simulink model "RmtAPP_ChkSig"  (R2016b)
settings: configuration reference "CodeGenConfigSet" (kept outside this file)
values from neighbouring files (symbols this model uses):
  RmtAPP_drLimNeg_C = Calibration.Parameter    [init_RmtAPP_ChkSig.m]    (also in init_RmtAPP_ChkSig_SIL.m = Simulink.Parameter)
  RmtAPP_drLimpMax_C = Calibration.Parameter    [init_RmtAPP_ChkSig.m]    (also in init_RmtAPP_ChkSig_SIL.m = Simulink.Parameter)
  RmtAPP_drLimPos_C = Calibration.Parameter    [init_RmtAPP_ChkSig.m]    (also in init_RmtAPP_ChkSig_SIL.m = Simulink.Parameter)
  RmtAPP_rLimpMax_C = Calibration.Parameter    [init_RmtAPP_ChkSig.m]    (also in init_RmtAPP_ChkSig_SIL.m = Simulink.Parameter)
  RmtAPP_rPlaMaxVal_C = Calibration.Parameter    [init_RmtAPP_ChkSig.m]    (also in init_RmtAPP_ChkSig_SIL.m = Simulink.Parameter)
  RmtAPP_rThresAliveDet_C = Calibration.Parameter    [init_RmtAPP_ChkSig.m]    (also in init_RmtAPP_ChkSig_SIL.m = Simulink.Parameter)
  RmtAPP_swtAliveDetEna_C = Calibration.Parameter    [init_RmtAPP_ChkSig.m]    (also in init_RmtAPP_ChkSig_SIL.m = Simulink.Parameter)
  RmtAPP_swtPlaChkEna_C = Calibration.Parameter    [init_RmtAPP_ChkSig.m]    (also in init_RmtAPP_ChkSig_SIL.m = Simulink.Parameter)
  RmtAPP_tiAliveDebHiLo_C = Calibration.Parameter    [init_RmtAPP_ChkSig.m]    (also in init_RmtAPP_ChkSig_SIL.m = Simulink.Parameter)
  RmtAPP_tiAliveDebLoHi_C = Calibration.Parameter    [init_RmtAPP_ChkSig.m]    (also in init_RmtAPP_ChkSig_SIL.m = Simulink.Parameter)
undefined symbols (not defined in the file or in its folder): RmtAPP_ChkSig_DT, Switch_conv
libraries: CXLib x9
settings Model: Creator=bianxuyin  LastModifiedBy=bianxuyin
settings ConfigSetRef: SourceLocation=Base Workspace

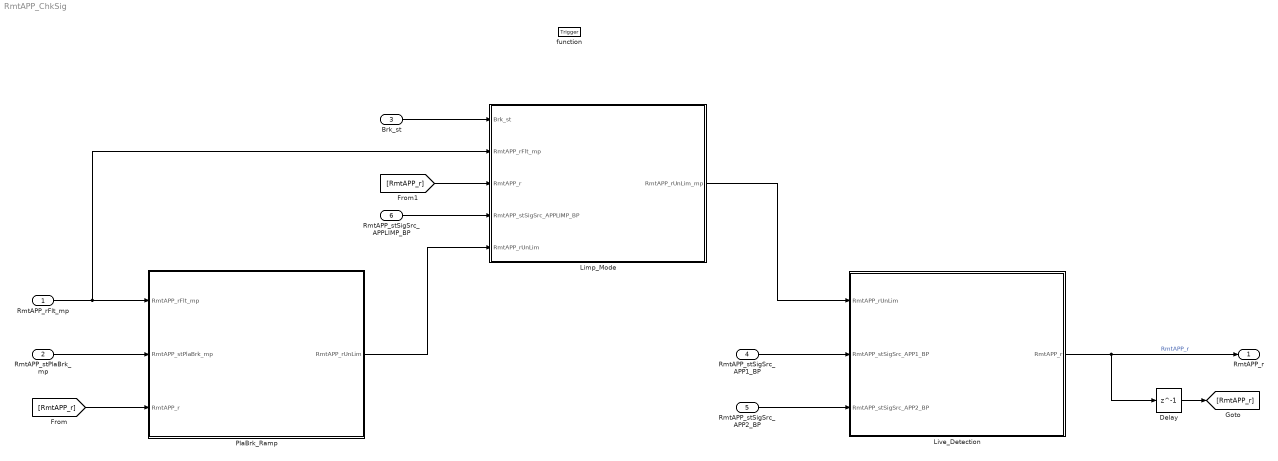
== system RmtAPP_ChkSig ==
  RmtAPP_rFlt_mp : Inport  Tag=%  Description=Remote Acceleration pedal position filtered value  OutMin=0  OutMax=100  OutDataTypeStr=Accpedal_rate
  RmtAPP_stPlaBrk_mp : Inport  Description=State of plausibility RmtAPP with brake  Port=2  OutMin=0  OutMax=1  OutDataTypeStr=boolean
  Brk_st : Inport  Description=Brake switch state  Port=3  OutMin=0  OutMax=255  OutDataTypeStr=State_uint8
  RmtAPP_stSigSrc_APP1_BP : Inport  Description=Sensor 1 is the reference variable, Sensor 2 value is defective  Port=4  OutMin=0  OutMax=1  OutDataTypeStr=boolean
  RmtAPP_stSigSrc_APP2_BP : Inport  Description=Sensor 2 is the reference variable,Sensor1 value is defective  Port=5  OutMin=0  OutMax=1  OutDataTypeStr=boolean
  RmtAPP_stSigSrc_APPLIMP_BP : Inport  Description=Substitute operation active, remote accelerator pedal sensor value and accelerator pedal sensor increase are limited  Port=6  OutMin=0  OutMax=1  OutDataTypeStr=boolean
  function : TriggerPort  TriggerType=function-call  VariantControl=Variant
  Delay : Delay  DelayLength=1  InitialCondition=0
  Limp_Mode : Subsystem
  Live_Detection : Subsystem
  PlaBrk_Ramp : Subsystem
  RmtAPP_r : Outport  Tag=%  Description=Remote Acceleration pedal sensor 1 value after fault handling  OutMin=0  OutMax=100  OutDataTypeStr=Accpedal_rate
  wires:
  Brk_st/1 -> Limp_Mode/1(Brk_st)
  RmtAPP_stSigSrc_APPLIMP_BP/1 -> Limp_Mode/4(RmtAPP_stSigSrc_APPLIMP_BP)
  Limp_Mode/1(RmtAPP_rUnLim_mp) -> Live_Detection/1(RmtAPP_rUnLim)
  RmtAPP_stSigSrc_APP1_BP/1 -> Live_Detection/2(RmtAPP_stSigSrc_APP1_BP)
  RmtAPP_stSigSrc_APP2_BP/1 -> Live_Detection/3(RmtAPP_stSigSrc_APP2_BP)
  Live_Detection/1(RmtAPP_r) -> Delay/1, RmtAPP_r/1  "RmtAPP_r"
  PlaBrk_Ramp/1(RmtAPP_rUnLim) -> Limp_Mode/5(RmtAPP_rUnLim)
  RmtAPP_rFlt_mp/1 -> Limp_Mode/2(RmtAPP_rFlt_mp), PlaBrk_Ramp/1(RmtAPP_rFlt_mp)
  RmtAPP_stPlaBrk_mp/1 -> PlaBrk_Ramp/2(RmtAPP_stPlaBrk_mp)
  Delay/1 -> [RmtAPP_r]
  [RmtAPP_r] -> PlaBrk_Ramp/3(RmtAPP_r)
  [RmtAPP_r] -> Limp_Mode/3(RmtAPP_r)

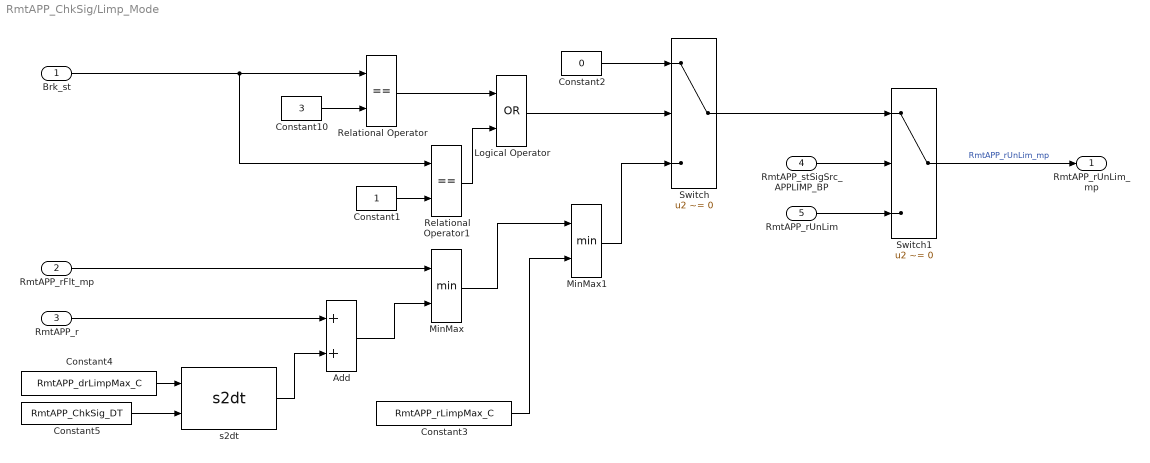
== system RmtAPP_ChkSig/Limp_Mode ==
  Brk_st : Inport  Description=Brake switch state  OutMin=0  OutMax=255
  RmtAPP_rFlt_mp : Inport  Tag=%  Description=Remote Acceleration pedal position filtered value  Port=2  OutMin=0  OutMax=100
  RmtAPP_r : Inport  Tag=%  Description=Remote Acceleration pedal position filtered value  Port=3  OutMin=0  OutMax=100
  RmtAPP_stSigSrc_APPLIMP_BP : Inport  Description=Substitute operation active, remote accelerator pedal sensor value and accelerator pedal sensor increase are limited  Port=4  OutMin=0  OutMax=1
  RmtAPP_rUnLim : Inport  Tag=%  Description=Remote Acceleration pedal position filtered value  Port=5  OutMin=0  OutMax=100
  Add : Sum  InputSameDT=on
  Constant1 : Constant  OutDataTypeStr=Inherit: Inherit via back propagation
  Constant10 : Constant  Value=3  OutDataTypeStr=Inherit: Inherit via back propagation
  Constant2 : Constant  Value=0  OutDataTypeStr=Inherit: Inherit via back propagation
  Constant3 : Constant  Value=RmtAPP_rLimpMax_C
  Constant4 : Constant  Value=RmtAPP_drLimpMax_C
  Constant5 : Constant  Value=RmtAPP_ChkSig_DT
  Logical Operator : Logic  Operator=OR  AllPortsSameDT=off  OutDataTypeStr=boolean
  MinMax : MinMax  Inputs=2  InputSameDT=on
  MinMax1 : MinMax  Inputs=2  InputSameDT=on
  Relational Operator : RelationalOperator  Operator===  OutDataTypeStr=boolean  RndMeth=Simplest
  Relational Operator1 : RelationalOperator  Operator===  OutDataTypeStr=boolean  RndMeth=Simplest
  Switch : Switch  Criteria=u2 ~= 0
  Switch1 : Switch  Criteria=u2 ~= 0
  s2dt : CXLib/s2dt
  RmtAPP_rUnLim_mp : Outport  Tag=%  Description=Remote Acceleration pedal sensor 1 value after fault handling  OutMin=0  OutMax=100  OutDataTypeStr=Accpedal_rate
  wires:
  Brk_st/1 -> Relational Operator1/1, Relational Operator/1
  Constant10/1 -> Relational Operator/2
  Relational Operator/1 -> Logical Operator/1
  Relational Operator1/1 -> Logical Operator/2
  Constant1/1 -> Relational Operator1/2
  Logical Operator/1 -> Switch/2
  Constant2/1 -> Switch/1
  MinMax/1 -> MinMax1/1
  MinMax1/1 -> Switch/3
  Constant3/1 -> MinMax1/2
  Add/1 -> MinMax/2
  RmtAPP_r/1 -> Add/1
  RmtAPP_rFlt_mp/1 -> MinMax/1
  s2dt/1 -> Add/2
  Constant4/1 -> s2dt/1
  Constant5/1 -> s2dt/2
  Switch/1 -> Switch1/1
  RmtAPP_stSigSrc_APPLIMP_BP/1 -> Switch1/2
  RmtAPP_rUnLim/1 -> Switch1/3
  Switch1/1 -> RmtAPP_rUnLim_mp/1  "RmtAPP_rUnLim_mp"

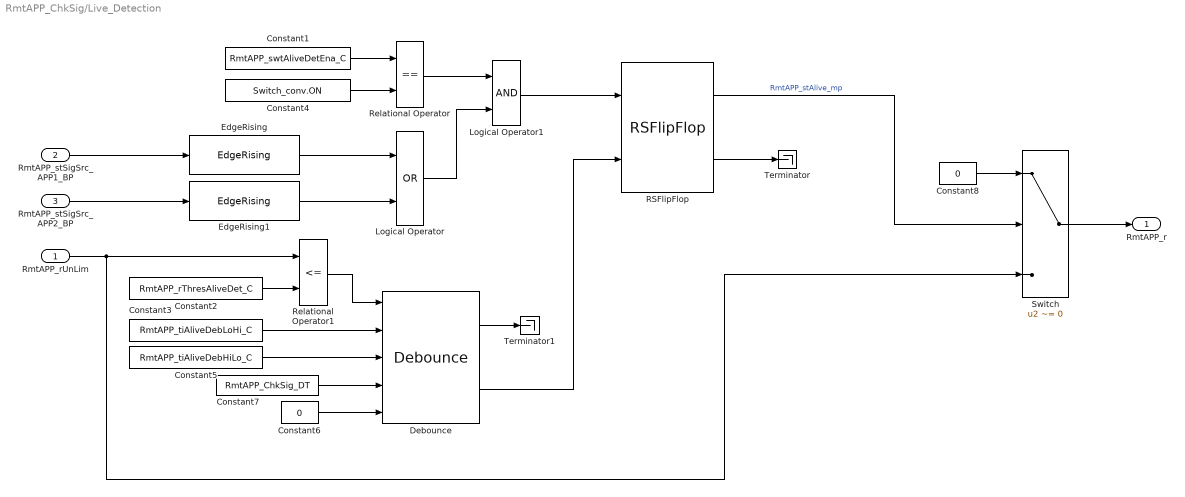
== system RmtAPP_ChkSig/Live_Detection ==
  RmtAPP_rUnLim : Inport  Description=Sensor 1 is the reference variable, Sensor 2 value is defective  OutMin=0  OutMax=1  OutDataTypeStr=Accpedal_rate
  RmtAPP_stSigSrc_APP1_BP : Inport  Description=Sensor 1 is the reference variable, Sensor 2 value is defective  Port=2  OutMin=0  OutMax=1  OutDataTypeStr=boolean
  RmtAPP_stSigSrc_APP2_BP : Inport  Description=Sensor 2 is the reference variable,Sensor1 value is defective  Port=3  OutMin=0  OutMax=1  OutDataTypeStr=boolean
  Constant1 : Constant  Value=RmtAPP_swtAliveDetEna_C
  Constant2 : Constant  Value=RmtAPP_rThresAliveDet_C
  Constant3 : Constant  Value=RmtAPP_tiAliveDebLoHi_C
  Constant4 : Constant  Value=Switch_conv.ON  OutDataTypeStr=Inherit: Inherit via back propagation
  Constant5 : Constant  Value=RmtAPP_tiAliveDebHiLo_C
  Constant6 : Constant  Value=0  OutDataTypeStr=Inherit: Inherit via back propagation
  Constant7 : Constant  Value=RmtAPP_ChkSig_DT  OutDataTypeStr=Inherit: Inherit via back propagation
  Constant8 : Constant  Value=0  OutDataTypeStr=Inherit: Inherit via back propagation
  Debounce : CXLib/Debounce
  EdgeRising : CXLib/EdgeRising
  EdgeRising1 : CXLib/EdgeRising
  Logical Operator : Logic  Operator=OR  OutDataTypeStr=boolean
  Logical Operator1 : Logic  OutDataTypeStr=boolean
  RSFlipFlop : CXLib/RSFlipFlop
  Relational Operator : RelationalOperator  Operator===  OutDataTypeStr=boolean  RndMeth=Simplest  InputSameDT=on
  Relational Operator1 : RelationalOperator  Operator=<=  OutDataTypeStr=boolean  RndMeth=Simplest  InputSameDT=on
  Switch : Switch  Criteria=u2 ~= 0
  Terminator : Terminator
  Terminator1 : Terminator
  RmtAPP_r : Outport  Tag=%  Description=Remote Acceleration pedal sensor 1 value after fault handling  OutMin=0  OutMax=100  OutDataTypeStr=Accpedal_rate
  wires:
  RmtAPP_stSigSrc_APP1_BP/1 -> EdgeRising/1
  Constant4/1 -> Relational Operator/2
  Constant1/1 -> Relational Operator/1
  Relational Operator/1 -> Logical Operator1/1
  Logical Operator/1 -> Logical Operator1/2
  Logical Operator1/1 -> RSFlipFlop/1
  RSFlipFlop/2 -> Terminator/1
  Debounce/1 -> Terminator1/1
  Debounce/2 -> RSFlipFlop/2
  Relational Operator1/1 -> Debounce/1
  RmtAPP_rUnLim/1 -> Relational Operator1/1, Switch/3
  Constant2/1 -> Relational Operator1/2
  Constant3/1 -> Debounce/2
  Constant5/1 -> Debounce/3
  Constant6/1 -> Debounce/5
  Constant7/1 -> Debounce/4
  RSFlipFlop/1 -> Switch/2  "RmtAPP_stAlive_mp"
  Constant8/1 -> Switch/1
  Switch/1 -> RmtAPP_r/1
  EdgeRising/1 -> Logical Operator/1
  RmtAPP_stSigSrc_APP2_BP/1 -> EdgeRising1/1
  EdgeRising1/1 -> Logical Operator/2

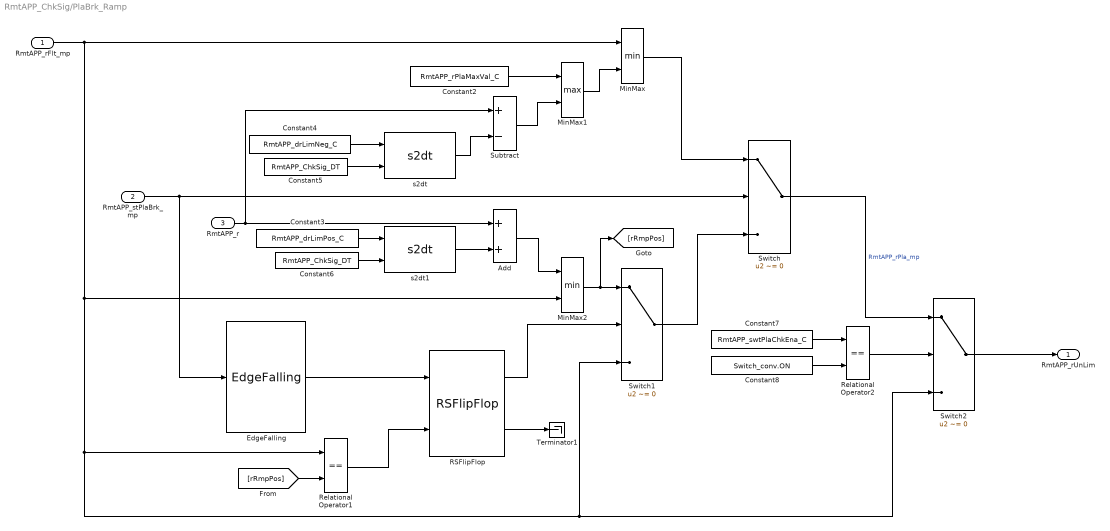
== system RmtAPP_ChkSig/PlaBrk_Ramp ==
  RmtAPP_rFlt_mp : Inport  Tag=%  Description=Remote Acceleration pedal position filtered value  OutMin=0  OutMax=100
  RmtAPP_stPlaBrk_mp : Inport  Description=State of plausibility RmtAPP with brake  Port=2  OutMin=0  OutMax=1
  RmtAPP_r : Inport  Description=State of plausibility RmtAPP with brake  Port=3  OutMin=0  OutMax=1
  Add : Sum  InputSameDT=on
  Constant2 : Constant  Value=RmtAPP_rPlaMaxVal_C
  Constant3 : Constant  Value=RmtAPP_drLimPos_C
  Constant4 : Constant  Value=RmtAPP_drLimNeg_C  VectorParams1D=off
  Constant5 : Constant  Value=RmtAPP_ChkSig_DT  OutDataTypeStr=Inherit: Inherit via back propagation
  Constant6 : Constant  Value=RmtAPP_ChkSig_DT  OutDataTypeStr=Inherit: Inherit via back propagation
  Constant7 : Constant  Value=RmtAPP_swtPlaChkEna_C
  Constant8 : Constant  Value=Switch_conv.ON  OutDataTypeStr=Inherit: Inherit via back propagation
  EdgeFalling : CXLib/EdgeFalling
  MinMax : MinMax  Inputs=2  InputSameDT=on
  MinMax1 : MinMax  Function=max  Inputs=2  InputSameDT=on
  MinMax2 : MinMax  Inputs=2  InputSameDT=on
  RSFlipFlop : CXLib/RSFlipFlop
  Relational Operator1 : RelationalOperator  Operator===  OutDataTypeStr=boolean  RndMeth=Simplest
  Relational Operator2 : RelationalOperator  Operator===  OutDataTypeStr=boolean  RndMeth=Simplest
  Subtract : Sum  Inputs=+-  InputSameDT=on
  Switch : Switch  Criteria=u2 ~= 0
  Switch1 : Switch  Criteria=u2 ~= 0
  Switch2 : Switch  Criteria=u2 ~= 0
  Terminator1 : Terminator
  s2dt : CXLib/s2dt
  s2dt1 : CXLib/s2dt
  RmtAPP_rUnLim : Outport  Tag=%  Description=Remote Acceleration pedal sensor 1 value after fault handling  OutMin=0  OutMax=100  OutDataTypeStr=Accpedal_rate
  wires:
  Subtract/1 -> MinMax1/2
  Constant2/1 -> MinMax1/1
  MinMax1/1 -> MinMax/2
  RmtAPP_rFlt_mp/1 -> MinMax2/2, Switch1/3, Switch2/3, Relational Operator1/1, MinMax/1
  RmtAPP_stPlaBrk_mp/1 -> EdgeFalling/1, Switch/2
  MinMax/1 -> Switch/1
  RmtAPP_r/1 -> Add/1, Subtract/1
  Add/1 -> MinMax2/1
  MinMax2/1 -> [rRmpPos], Switch1/1
  Switch1/1 -> Switch/3
  RSFlipFlop/1 -> Switch1/2
  RSFlipFlop/2 -> Terminator1/1
  EdgeFalling/1 -> RSFlipFlop/1
  Relational Operator1/1 -> RSFlipFlop/2
  s2dt1/1 -> Add/2
  Constant3/1 -> s2dt1/1
  Constant6/1 -> s2dt1/2
  Switch/1 -> Switch2/1  "RmtAPP_rPla_mp"
  Relational Operator2/1 -> Switch2/2
  Constant7/1 -> Relational Operator2/1
  Constant8/1 -> Relational Operator2/2
  [rRmpPos] -> Relational Operator1/2
  Switch2/1 -> RmtAPP_rUnLim/1
  Constant4/1 -> s2dt/1
  Constant5/1 -> s2dt/2
  s2dt/1 -> Subtract/2
